simulink model "normalControl"  (R2019a)
settings: Solver=VariableStepDiscrete  StartTime=0.0  StopTime=0  RelTol=1e-3
values from neighbouring files (symbols this model uses):
  curvature = zeros(predHorizon, 1)    [curv.m]
  latDev = 0    [matlab.mat]
  timeSample = 0.2    [matlab.mat]    (also in param.mat = 0.1)
  Vx = 1    [matlab.mat]
  yawDev = atan(df_init)    [curv.m]    (also in matlab.mat = 0)
libraries: mpcadaslib x1
settings Model: ExtModeTrigDuration=100  Creator=Daniel Galhoz  LastModifiedBy=Daniel Galhoz
settings SolverCC: DecoupledContinuousIntegration=on  MinimalZcImpactIntegration=on
settings DataIOCC: SaveOutput=off  StateSaveName=tmp_raccel_xout  SignalLoggingName=tmp_raccel_logsout
settings OptimizationCC: EfficientMapNaN2IntZero=off
settings DebuggingCC: ReadBeforeWriteMsg=DisableAll  WriteAfterWriteMsg=DisableAll  WriteAfterReadMsg=DisableAll  MultiTaskDSMMsg=none
settings HardwareCC: TargetBitPerPointer=64  TargetBitPerSizeT=64  TargetBitPerPtrDiffT=64  TargetLongLongMode=on  TargetIntDivRoundTo=Zero  TargetEndianess=LittleEndian  TargetWordSize=64  TargetHWDeviceType=MATLAB Host  ProdEqTarget=off
settings ModelReferenceCC: UpdateModelReferenceTargets=IfOutOfDate
settings SFSimCC: SFSimEcho=off
settings RTWCC: SystemTargetFile=raccel.tlc  TemplateMakefile=raccel_default_tmf  RTWVerbose=off  RTWUseSimCustomCode=on
settings CodeAppCC: GenerateComments=off  MaxIdLength=128
settings RaccelTargetCC: GeneratePreprocessorConditionals=Use local settings  MultiInstanceERTCode=off  PreserveStateflowLocalDataDimensions=off  ENABLE_SLEXEC_SSBRIDGE=1  RTWCAPIParams=on

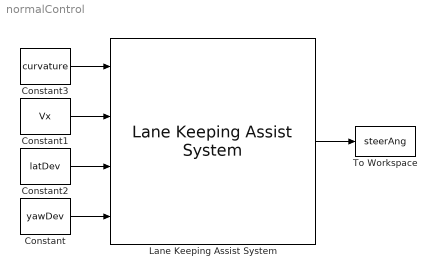
== system normalControl ==
  Constant : Constant  Value=yawDev  OutDataTypeStr=double
  Constant1 : Constant  Value=Vx  OutDataTypeStr=double
  Constant2 : Constant  Value=latDev  OutDataTypeStr=double
  Constant3 : Constant  Value=curvature  OutDataTypeStr=double
  Lane Keeping Assist System : mpcadaslib/Lane Keeping Assist System  ModelType=Use vehicle parameters  VehicleMass=mass  VehicleYawInertia=Iyam  LengthToFront=Lf  LengthToRear=Lr  FrontTireStiffness=Cf  RearTireStiffness=Cr  EgoModelMatrixA=[-4.4021 ,-12.4603;1.3913,-5.1868]  EgoModelMatrixB=[24.1270;15.8609]  EgoModelMatrixC=[1,0;0,1]  InitialLongVel=Vx  TransportLag=0  MinSteering=minStAng  umin_ext=off  MaxSteering=maxStAng  umax_ext=off  Ts=timeSample  PredictionHorizon=predHorizon  ControllerBehavior=controlBehavior  suboptimal=off  maxiter=10  datatypeopt=single  optmode=off  trackmode=off
      settings: SourceProductName=MATLAB Runtime - Model Predictive Control Toolbox Addin  SourceProductBaseCode=Missing
  To Workspace : ToWorkspace  VariableName=steerAng  SampleTime=-1
      settings: MaxDataPoints=1
  wires:
  Lane Keeping Assist System/1 -> To Workspace/1
  Constant1/1 -> Lane Keeping Assist System/2
  Constant2/1 -> Lane Keeping Assist System/3
  Constant3/1 -> Lane Keeping Assist System/1
  Constant/1 -> Lane Keeping Assist System/4
